simulink model "pompa"  (R2017b)
settings: Solver=VariableStepAuto  StartTime=0.0  StopTime=10.0  RelTol=1e-3
values from neighbouring files (symbols this model uses):
  k11 = k2^2+4*(k-k3)*k1    (= 0.0890826)    [modelare.m]
  k12 = 4*(k-k3)*2    (= 0.2848)    [modelare.m]
  k13 = 2*(k-k3)    (= 0.0712)    [modelare.m]
  k2 = -0.015    [modelare.m]
settings Model: Creator=alinvoicu26  LastModifiedBy=alinvoicu26

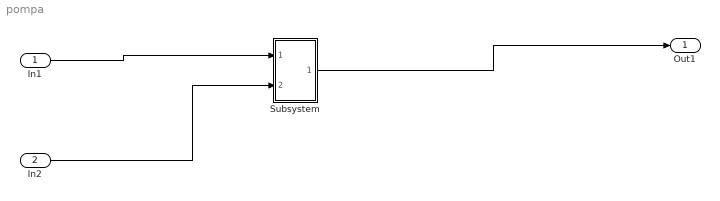
== system pompa ==
  In1 : Inport
  In2 : Inport  Port=2
  Subsystem : Subsystem
  Out1 : Outport
  wires:
  In1/1 -> Subsystem/1(In1)
  In2/1 -> Subsystem/2(In2)
  Subsystem/1(Out1) -> Out1/1

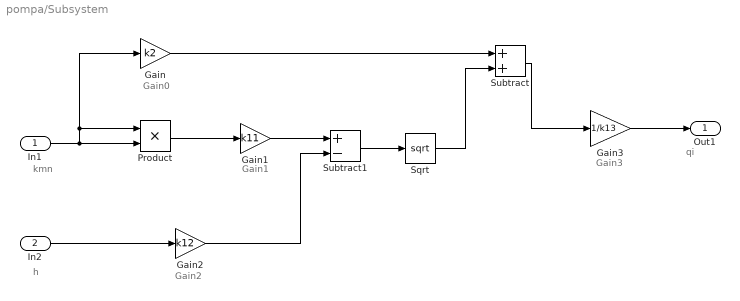
== system pompa/Subsystem ==
  note: Gain3
  note: Gain0
  note: Gain2
  note: Gain1
  note: qi
  note: h
  note: kmn
  In1 : Inport
  In2 : Inport  Port=2
  Gain : Gain  Gain=k2
  Gain1 : Gain  Gain=k11
  Gain2 : Gain  Gain=k12
  Gain3 : Gain  Gain=1/k13
  Product : Product
  Sqrt : Sqrt  SaturateOnIntegerOverflow=on
  Subtract : Sum
  Subtract1 : Sum  Inputs=+-
  Out1 : Outport
  wires:
  In1/1 -> Product/1, Gain/1, Product/2
  Product/1 -> Gain1/1
  Sqrt/1 -> Subtract/2
  Gain/1 -> Subtract/1
  Subtract/1 -> Gain3/1
  Gain2/1 -> Subtract1/2
  Gain1/1 -> Subtract1/1
  Gain3/1 -> Out1/1
  Subtract1/1 -> Sqrt/1
  In2/1 -> Gain2/1
